simulink model "Rotor_Dynamic_Inflow"  (R2022b)
settings: Solver=VariableStepAuto  StartTime=0.0  StopTime=8  MaxStep=.0001  RelTol=1e-3
InitFcn:
  | dir = pwd; %model directory
  | 
  | %go to look up tables
  | cd('../Look Up Tables') %look up table directory
  | 
  | %Ct, Cp, and theta of rotor
  | load('BEMTdata_coax_final.mat');
  | 
  | %Peters-He model parameters (M,L,shape)
  | load('PetersHe_1state.mat');
  | 
  | %go back to model directory
  | cd(pwd);
  | 
  | %rotor parameters
  | d_prop = 2*1.016;
  | R_c = d_prop/2*.12;
  | Nb = 2;
  | dr = rotor_params.dr;
  | Inertia = rotor_params.I_rotor;
  | kappa = rotor_params.kappa;
  | 
  | %atmospheric properties
  | rho_air = 1.225;
  | 
  | %model conditions
  | RPM0 = 942;
  | RPMf = 972;
  | ramp = 3000; %[rpm/s]
  | k = 0.865; %mass flow correction
  | shape = model.psi_a(1);
  | 
  | cd(dir)
values from neighbouring files (symbols this model uses):
  Cp = [0.000195201118563 0.000195344815163 0.000195970524669 0.000196911243155 0.000198292722473 0.000199793715635 0.000201836164013 0.000204359459521 0.00020706119236 0.00020992934584 0.000212955219574 0.000216131124695 ... (150 elements, 1x150)]    [BEMT-1.mat]    (also in BEMT-2.mat = [5.908e-05 5.908e-05 5.908e-05 5.908e-05 5.908e-05 5.908e-05; BEMT-3.mat = [6.167e-05 6.167e-05 6.167e-05 6.167e-05 6.167e-05 6.1671725; BEMT-PF-Isolated-1.mat = [6.88284627296e-05 6.76929537705e-05 6.92283244838e-05 7.518; BEMT-PF-Isolated-2.mat = [6.88286203447e-05 6.76929720507e-05 6.92293837373e-05 7.518)
  Ct = [0 8.42066058624e-05 0.000168413211725 0.000252619817587 0.000348569118235 0.000435711397794 0.000522853677352 0.000609995956911 0.00069713823647 0.000784280516029 0.000871422795587 0.000958565075146 ... (150 elements, 1x150)]    [BEMT-1.mat]    (also in BEMT-2.mat = [-0.000241284312952 -0.00019885713846 -0.000156429963968 -0.; BEMT-3.mat = [-0.000252881464423 -0.00020500571035 -0.00015767832519 -0.0; BEMT-PF-Isolated-1.mat = [-0.000124730397385 6.78902114512e-07 0.000152796242494 0.00; BEMT-PF-Isolated-2.mat = [-0.000124743531158 6.68801957239e-07 0.000152879013625 0.00)
  model =     [DynInflow-1.mat]    (also in PP-1.mat; PP-2.mat; PP-3.mat)
  rotor_params =     [DynInflow-1.mat]    (also in PP-1.mat; PP-2.mat; PP-3.mat)
  theta = [-1.24244156171 -0.730247869575 -0.489791195362 -0.291308360013 -0.0904887039498 0.0775201787218 0.236938510902 0.389966557012 0.537998944025 0.680941129328 0.820002111662 0.955737387113 ... (150 elements, 1x150)]    [BEMT-1.mat]    (also in BEMT-2.mat = [-2.67472972391 -2.52181622329 -2.35655527709 -2.17339529035; BEMT-3.mat = [-2.61565298703 -2.45920727031 -2.29202818901 -2.11251263407; BEMT-PF-Isolated-1.mat = [-2 -1 0 1 2 3 4 5 6 7 8 9 ... (16 elements, 1x16)]; BEMT-PF-Isolated-2.mat = [-2 -1 0 1 2 3 4 5 6 7 8 9 ... (16 elements, 1x16)])
settings Model: PacingRate=0.110000  Creator=msa2925  LastModifiedBy=asper101

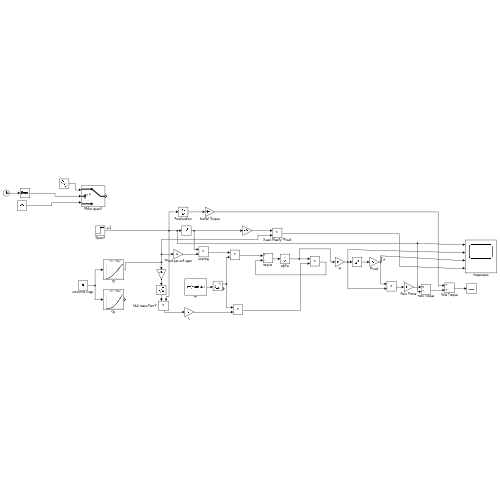
[thumbnail: Simulink's stored preview of the top-level diagram]
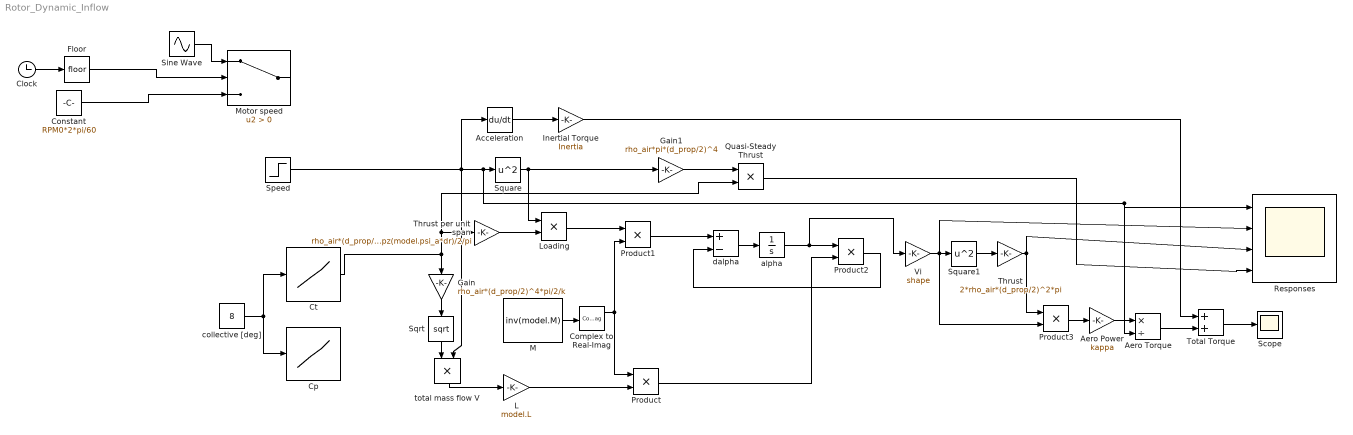
== system Rotor_Dynamic_Inflow ==
  Acceleration : Derivative
  Aero Power : Gain  Gain=kappa
  Aero Torque : Product  Inputs=*/
  Clock : Clock
  Complex to Real-Imag : ComplexToRealImag
  Constant : Constant  Value=RPM0*2*pi/60
  Cp : Lookup_n-D  NumberOfTableDimensions=1  BreakpointsForDimension1=theta  BreakpointsForDimension2=[1:3]  Table=Cp  InternalRulePriority=Speed  RndMeth=Simplest
  Ct : Lookup_n-D  NumberOfTableDimensions=1  BreakpointsForDimension1=theta  BreakpointsForDimension2=[1:3]  Table=Ct  InternalRulePriority=Speed  RndMeth=Simplest
  Floor : Rounding
  Gain : Gain  Gain=rho_air*(d_prop/2)^4*pi/2/k
  Gain1 : Gain  Gain=rho_air*pi*(d_prop/2)^4
  Inertial Torque : Gain  Gain=Inertia
  L : Gain  Gain=model.L
  Loading : Product
  M : Constant  Value=inv(model.M)
  Motor speed : Switch  Criteria=u2 > Threshold  SaturateOnIntegerOverflow=off  InputSameDT=off
  Product{,1..3} (4 alike) : Product
  Quasi-Steady Thrust : Product
  Responses : Scope  NumInputPorts=4
  Scope : Scope
  Sine Wave : Sin  Amplitude=30*2*pi/60  Bias=RPM0*2*pi/60  Frequency=4*2*pi  SampleTime=0
  Speed : Step  Time=3  Before=RPM0*2*pi/60  After=RPMf*2*pi/60  SampleTime=0
  Sqrt : Sqrt
  Square : Math  Operator=square
  Square1 : Math  Operator=square
  Thrust : Gain  Gain=2*rho_air*(d_prop/2)^2*pi
  Thrust per unit span : Gain  Gain=rho_air*(d_prop/2)^4*pi/(d_prop/2)*trapz(model.psi_a*dr)/2/pi
  Total Torque : Sum
  Vi : Gain  Gain=shape
  alpha : Integrator
  collective [deg] : Constant  Value=8
  dalpha : Sum  Inputs=+-
  total mass flow V : Product
  wires:
  collective [deg]/1 -> Cp/1, Ct/1
  Square/1 -> Gain1/1, Loading/1
  Loading/1 -> Product1/1
  Product1/1 -> dalpha/1
  alpha/1 -> Vi/1, Product2/1
  Product2/1 -> dalpha/2
  Gain/1 -> Sqrt/1
  Sqrt/1 -> total mass flow V/1
  total mass flow V/1 -> L/1
  L/1 -> Product/2
  Speed/1 -> Acceleration/1, Aero Torque/2, Responses/1, Square/1, total mass flow V/2
  Square1/1 -> Thrust/1
  Thrust/1 -> Product3/1, Responses/3
  Product/1 -> Product2/2
  dalpha/1 -> alpha/1
  Vi/1 -> Product3/2, Responses/2, Square1/1
  Thrust per unit span/1 -> Loading/2
  M/1 -> Complex to Real-Imag/1
  Complex to Real-Imag/1 -> Product1/2, Product/1
  Ct/1 -> Quasi-Steady Thrust/2, Thrust per unit span/1, Gain/1
  Product3/1 -> Aero Power/1
  Aero Power/1 -> Aero Torque/1
  Aero Torque/1 -> Total Torque/2
  Inertial Torque/1 -> Total Torque/1
  Sine Wave/1 -> Motor speed/1
  Floor/1 -> Motor speed/2
  Clock/1 -> Floor/1
  Constant/1 -> Motor speed/3
  Gain1/1 -> Quasi-Steady Thrust/1
  Quasi-Steady Thrust/1 -> Responses/4
  Total Torque/1 -> Scope/1
  Acceleration/1 -> Inertial Torque/1
